simulink model "main_simulink"  (R2014b)
settings: Solver=ode45  StartTime=0.0  StopTime=10.0  RelTol=1e-3
values from neighbouring files (symbols this model uses):
  init_state = [0 0 3 0 0 0 0 0 0 0 0 0]    [main.m]
settings Model: Creator=shuoli  LastModifiedBy=shuoli

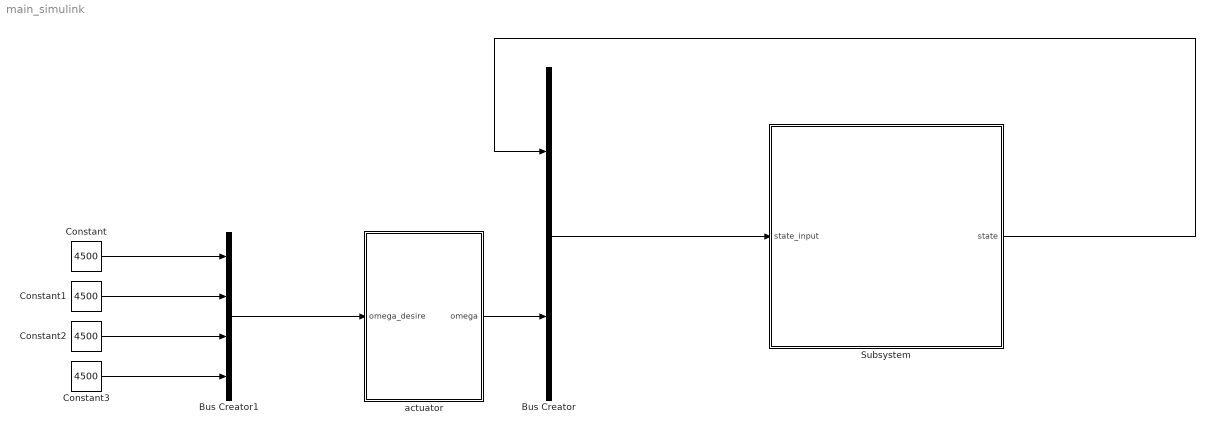
== system main_simulink ==
  Bus Creator : BusCreator  Inputs=2
  Bus Creator1 : BusCreator
  Constant{,1..3} (4 alike) : Constant  Value=4500
  Subsystem : Subsystem
  actuator : Subsystem
  wires:
  Constant/1 -> Bus Creator1/1
  Constant1/1 -> Bus Creator1/2
  Constant2/1 -> Bus Creator1/3
  Constant3/1 -> Bus Creator1/4
  Bus Creator/1 -> Subsystem/1(state_input)
  Subsystem/1(state) -> Bus Creator/1
  actuator/1(omega) -> Bus Creator/2
  Bus Creator1/1 -> actuator/1(omega_desire)

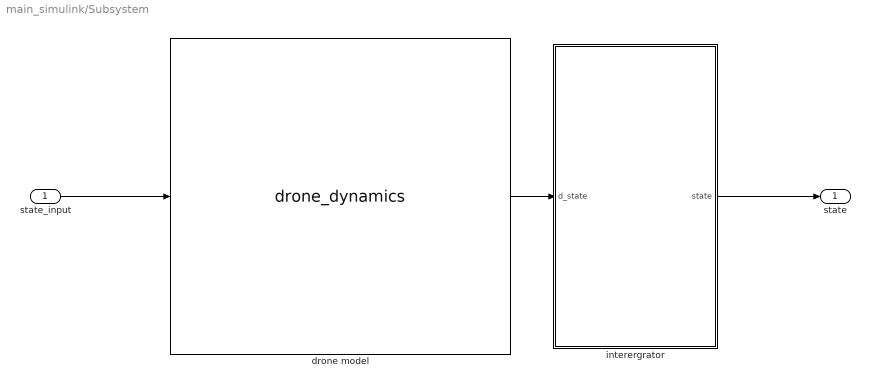
== system main_simulink/Subsystem ==
  state_input : Inport
  drone model : MATLABFcn  MATLABFcn=drone_dynamics
  interergrator : Subsystem
  state : Outport
  wires:
  state_input/1 -> drone model/1
  interergrator/1(state) -> state/1
  drone model/1 -> interergrator/1(d_state)

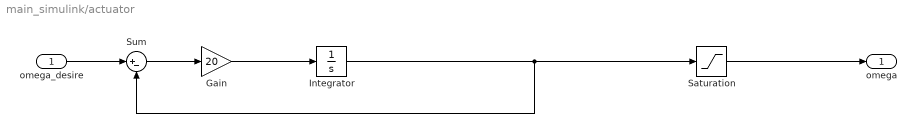
== system main_simulink/actuator ==
  omega_desire : Inport
  Gain : Gain  Gain=20
  Integrator : Integrator  InitialCondition=[4477,4477,4477,4477]
  Saturation : Saturate  UpperLimit=10000  LowerLimit=0
  Sum : Sum  Inputs=|+-
  omega : Outport
  wires:
  Integrator/1 -> Saturation/1, Sum/2
  omega_desire/1 -> Sum/1
  Sum/1 -> Gain/1
  Gain/1 -> Integrator/1
  Saturation/1 -> omega/1

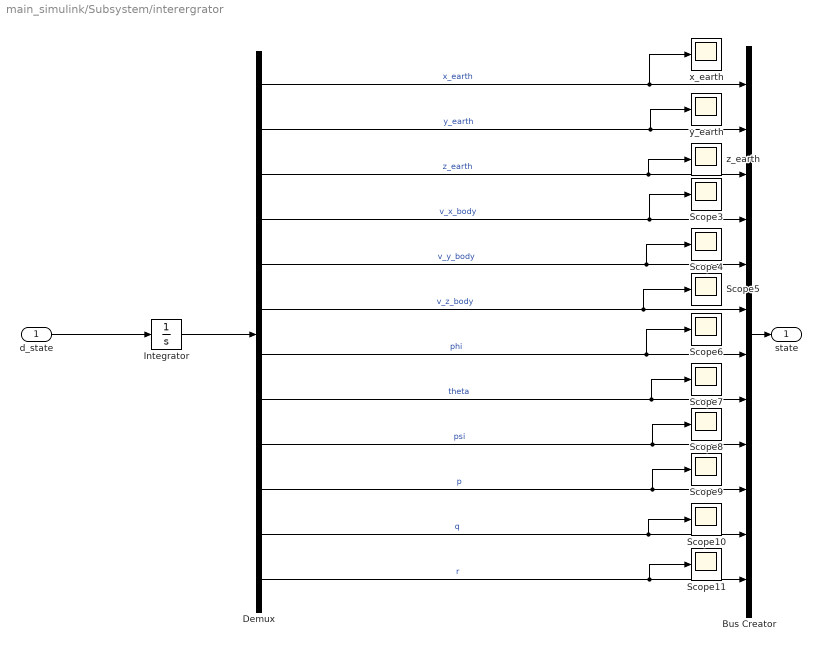
== system main_simulink/Subsystem/interergrator ==
  d_state : Inport
  Bus Creator : BusCreator  Inputs=12
  Demux : Demux  Outputs=12
  Integrator : Integrator  InitialCondition=init_state
  Scope{3..11} (9 alike) : Scope
      Scope10 settings: SaveName=ScopeData10
      Scope11 settings: SaveName=ScopeData11
      Scope3 settings: SaveName=ScopeData3
      Scope4 settings: SaveName=ScopeData4
      Scope5 settings: SaveName=ScopeData5
      Scope6 settings: SaveName=ScopeData6
      Scope7 settings: SaveName=ScopeData7
      Scope8 settings: SaveName=ScopeData8
      Scope9 settings: SaveName=ScopeData9
  x_earth : Scope
  y_earth : Scope
  z_earth : Scope
      settings: SaveName=ScopeData2
  state : Outport
  wires:
  Demux/8 -> Scope7/1, Bus Creator/8  "theta"
  Demux/12 -> Scope11/1, Bus Creator/12  "r"
  Demux/1 -> x_earth/1, Bus Creator/1  "x_earth"
  d_state/1 -> Integrator/1
  Demux/9 -> Scope8/1, Bus Creator/9  "psi"
  Demux/6 -> Scope5/1, Bus Creator/6  "v_z_body"
  Demux/7 -> Scope6/1, Bus Creator/7  "phi"
  Demux/4 -> Scope3/1, Bus Creator/4  "v_x_body"
  Demux/5 -> Scope4/1, Bus Creator/5  "v_y_body"
  Demux/2 -> y_earth/1, Bus Creator/2  "y_earth"
  Demux/10 -> Scope9/1, Bus Creator/10  "p"
  Demux/11 -> Scope10/1, Bus Creator/11  "q"
  Demux/3 -> z_earth/1, Bus Creator/3  "z_earth"
  Integrator/1 -> Demux/1
  Bus Creator/1 -> state/1
